simulink model "Q2_power_output"  (R2024b)
settings: Solver=VariableStepAuto  StartTime=0.0  StopTime=10.0  RelTol=1e-3
settings Model: Creator=Sagar  LastModifiedBy=Sagar

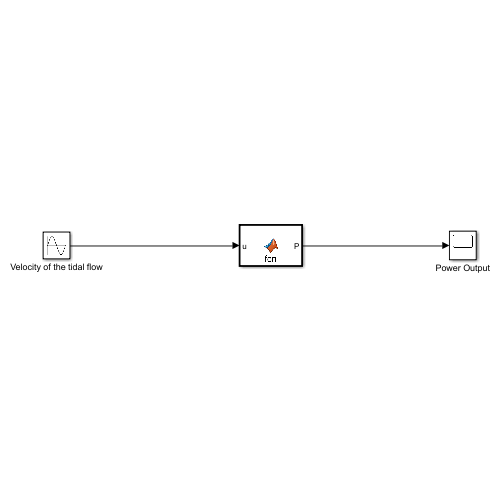
[thumbnail: Simulink's stored preview of the top-level diagram]
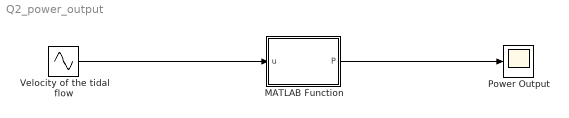
== system Q2_power_output ==
  MATLAB Function : MATLAB Function  TreatAsAtomicUnit=on
  Power Output : Scope
  Velocity of the tidal flow : Sin  SampleTime=0
  wires:
  Velocity of the tidal flow/1 -> MATLAB Function/1(u)
  MATLAB Function/1(P) -> Power Output/1

== matlab function Q2_power_output/MATLAB Function ==
  data: u input; P output
function P = fcn(u)
rho = 1025;
A = 100;
P = 0.5*rho*A*u*u*u;
